simulink model "AtmDcMotor"  (R2015a)
settings: configuration reference "SIMULATION_CONFIGURATION" (kept outside this file)
settings Model: CovSFcnEnable=off  Creator=moritz  LastModifiedBy=moritz
settings ConfigSetRef: SourceLocation=Base Workspace

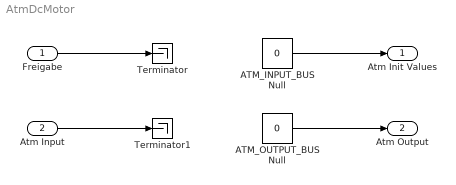
== system AtmDcMotor ==
  Freigabe : Inport  OutDataTypeStr=boolean
  Atm Input : Inport  Port=2  OutDataTypeStr=Bus: ATM_INPUT_BUS  BusOutputAsStruct=on
  ATM_INPUT_BUS Null : Constant  Value=0  OutDataTypeStr=Bus: ATM_INPUT_BUS  SampleTime=-1
  ATM_OUTPUT_BUS Null : Constant  Value=0  OutDataTypeStr=Bus: ATM_OUTPUT_BUS  SampleTime=-1
  Terminator : Terminator
  Terminator1 : Terminator
  Atm Init Values : Outport  OutDataTypeStr=Bus: ATM_INPUT_BUS  BusOutputAsStruct=on
  Atm Output : Outport  Port=2  OutDataTypeStr=Bus: ATM_OUTPUT_BUS  BusOutputAsStruct=on
  wires:
  Atm Input/1 -> Terminator1/1
  ATM_INPUT_BUS Null/1 -> Atm Init Values/1
  Freigabe/1 -> Terminator/1
  ATM_OUTPUT_BUS Null/1 -> Atm Output/1
